simulink library "lib_fuel_converter"  (Simulink 4.00)
undefined symbols (not defined in the file): acc_mech_eff, acc_mech_pwr, acc_mech_trq, air_cp, amb_tmp, cyc_mph, ex_gas_cp, fc_acc_mass, fc_base_mass, fc_c2i_th_cond, fc_c_init_tmp, fc_cl2h_eff, fc_CO2_to_FUELgps, fc_cold, fc_cold_tmp, fc_cp, fc_ct_trq, fc_emisv, fc_ext_sarea, fc_fuel_den, fc_fuel_lhv, fc_h2x_th_cond, fc_h_air_flow, fc_h_cp, fc_h_init_tmp, fc_hood_emisv, fc_hood_sarea, fc_i2x_th_cond, fc_i_init_tmp, fc_inertia, fc_map_spd, fc_map_trq, fc_max_trq, fc_nn_model_name, fc_pwr_scale, fc_spd_scale, fc_trq_scale, fc_tstat, fc_x_init_tmp, fd_ratio, gb_num_init, gb_ratio, pow, vc_idle_spd, vc_key_on, veh_glider_mass, veh_mass, wh_radius
libraries: lib_fuel_converter x6, lib_etc x4
(part 4 of 4)

== system lib_fuel_converter/configurable subsystems/fuel use and EO emis/fc temp correct/fc temp correct Variable Correction Factors (Map Based)/CO factor cold-to-hot ==
  x0 : Inport  Port=1  LatchInput=off
  y0 : Inport  Port=2  LatchInput=off
  Mux : Mux  Inputs=2
      settings: DisplayOption=none
  S-function : S-Function  FunctionName=sftable2  Parameters=xindex, yindex, table  PortCounts=[]  SFunctionModules=''
  table out : Outport  Port=1  InitialOutput=0
  wires:
  Mux/1 -> S-function/1
  x0/1 -> Mux/1
  S-function/1 -> table out/1
  y0/1 -> Mux/2

== system lib_fuel_converter/configurable subsystems/fuel use and EO emis/fc temp correct/fc temp correct Variable Correction Factors (Map Based)/HC factor cold-to-hot ==
  x0 : Inport  Port=1  LatchInput=off
  y0 : Inport  Port=2  LatchInput=off
  Mux : Mux  Inputs=2
      settings: DisplayOption=none
  S-function : S-Function  FunctionName=sftable2  Parameters=xindex, yindex, table  PortCounts=[]  SFunctionModules=''
  table out : Outport  Port=1  InitialOutput=0
  wires:
  Mux/1 -> S-function/1
  x0/1 -> Mux/1
  S-function/1 -> table out/1
  y0/1 -> Mux/2

== system lib_fuel_converter/configurable subsystems/fuel use and EO emis/fc temp correct/fc temp correct Variable Correction Factors (Map Based)/NOx factor cold-to-hot ==
  x0 : Inport  Port=1  LatchInput=off
  y0 : Inport  Port=2  LatchInput=off
  Mux : Mux  Inputs=2
      settings: DisplayOption=none
  S-function : S-Function  FunctionName=sftable2  Parameters=xindex, yindex, table  PortCounts=[]  SFunctionModules=''
  table out : Outport  Port=1  InitialOutput=0
  wires:
  Mux/1 -> S-function/1
  x0/1 -> Mux/1
  S-function/1 -> table out/1
  y0/1 -> Mux/2

== system lib_fuel_converter/configurable subsystems/fuel use and EO emis/fc temp correct/fc temp correct Variable Correction Factors (Map Based)/PM factor cold-to-hot ==
  x0 : Inport  Port=1  LatchInput=off
  y0 : Inport  Port=2  LatchInput=off
  Mux : Mux  Inputs=2
      settings: DisplayOption=none
  S-function : S-Function  FunctionName=sftable2  Parameters=xindex, yindex, table  PortCounts=[]  SFunctionModules=''
  table out : Outport  Port=1  InitialOutput=0
  wires:
  Mux/1 -> S-function/1
  x0/1 -> Mux/1
  S-function/1 -> table out/1
  y0/1 -> Mux/2

== system lib_fuel_converter/configurable subsystems/fuel use and EO emis/fc temp correct/fc temp correct Variable Correction Factors (Map Based)/fuel factor cold-to-hot ==
  x0 : Inport  Port=1  LatchInput=off
  y0 : Inport  Port=2  LatchInput=off
  Mux : Mux  Inputs=2
      settings: DisplayOption=none
  S-function : S-Function  FunctionName=sftable2  Parameters=xindex, yindex, table  PortCounts=[]  SFunctionModules=''
  table out : Outport  Port=1  InitialOutput=0
  wires:
  Mux/1 -> S-function/1
  x0/1 -> Mux/1
  S-function/1 -> table out/1
  y0/1 -> Mux/2

== system lib_fuel_converter/configurable subsystems/fuel use and EO emis Neural Network Model/fc temp/fc mass heat flow/Block NOTES ==
  note: FUEL CONVERTER MASS HEAT LOSS
      | This block models the heat loss from a fuel converter (such as an IC engine).
      | Convection (as a function of vehicle speed), radiation, and conduction effects are included.
      | Engine cylinder (c), interior (i), exterior (x) and hood (h)
      | heat flows are estimated based on the temperatures from the previous iteration.

== system lib_fuel_converter/configurable subsystems/fuel use and EO emis Neural Network Model/fc temp/old fc coolant  temp. (C)/Block NOTES ==
  note: This block computes engine coolant temperature,
      | assuming that it asymptotically approaches its maximum
      | temperature when the engine is on, and asymptotically
      | approaches the ambient temperature when the engine
      | is off.  Temperatue rise rate is assumed to be a function
      | only of current engine coolant temperature, and the fall
      | rate is also a function of vehicle speed and ambient temperature.
      | There is no dependence on engine load or speed.

== system lib_fuel_converter/configurable subsystems/fuel use and EO emis Neural Network Model/fc temp correct/fc temp correct Constant Correction Factors (Equation Based)/Block NOTES ==
  note: This block determines actual fuel use and engine-out emissions
      | given the fully hot values and the engine coolant temperature.
      | The correlations used here were developed at NREL using
      | Hot and Cold Engine data collected
      | at Oak Ridge National Laboratory.

== system lib_fuel_converter/configurable subsystems/fuel use and EO emis Neural Network Model/fc temp correct/fc temp correct Variable Correction Factors (Map Based)/CO factor cold-to-hot ==
  x0 : Inport  Port=1  LatchInput=off
  y0 : Inport  Port=2  LatchInput=off
  Mux : Mux  Inputs=2
      settings: DisplayOption=none
  S-function : S-Function  FunctionName=sftable2  Parameters=xindex, yindex, table  PortCounts=[]  SFunctionModules=''
  table out : Outport  Port=1  InitialOutput=0
  wires:
  Mux/1 -> S-function/1
  x0/1 -> Mux/1
  S-function/1 -> table out/1
  y0/1 -> Mux/2

== system lib_fuel_converter/configurable subsystems/fuel use and EO emis Neural Network Model/fc temp correct/fc temp correct Variable Correction Factors (Map Based)/HC factor cold-to-hot ==
  x0 : Inport  Port=1  LatchInput=off
  y0 : Inport  Port=2  LatchInput=off
  Mux : Mux  Inputs=2
      settings: DisplayOption=none
  S-function : S-Function  FunctionName=sftable2  Parameters=xindex, yindex, table  PortCounts=[]  SFunctionModules=''
  table out : Outport  Port=1  InitialOutput=0
  wires:
  Mux/1 -> S-function/1
  x0/1 -> Mux/1
  S-function/1 -> table out/1
  y0/1 -> Mux/2

== system lib_fuel_converter/configurable subsystems/fuel use and EO emis Neural Network Model/fc temp correct/fc temp correct Variable Correction Factors (Map Based)/NOx factor cold-to-hot ==
  x0 : Inport  Port=1  LatchInput=off
  y0 : Inport  Port=2  LatchInput=off
  Mux : Mux  Inputs=2
      settings: DisplayOption=none
  S-function : S-Function  FunctionName=sftable2  Parameters=xindex, yindex, table  PortCounts=[]  SFunctionModules=''
  table out : Outport  Port=1  InitialOutput=0
  wires:
  Mux/1 -> S-function/1
  x0/1 -> Mux/1
  S-function/1 -> table out/1
  y0/1 -> Mux/2

== system lib_fuel_converter/configurable subsystems/fuel use and EO emis Neural Network Model/fc temp correct/fc temp correct Variable Correction Factors (Map Based)/PM factor cold-to-hot ==
  x0 : Inport  Port=1  LatchInput=off
  y0 : Inport  Port=2  LatchInput=off
  Mux : Mux  Inputs=2
      settings: DisplayOption=none
  S-function : S-Function  FunctionName=sftable2  Parameters=xindex, yindex, table  PortCounts=[]  SFunctionModules=''
  table out : Outport  Port=1  InitialOutput=0
  wires:
  Mux/1 -> S-function/1
  x0/1 -> Mux/1
  S-function/1 -> table out/1
  y0/1 -> Mux/2

== system lib_fuel_converter/configurable subsystems/fuel use and EO emis Neural Network Model/fc temp correct/fc temp correct Variable Correction Factors (Map Based)/fuel factor cold-to-hot ==
  x0 : Inport  Port=1  LatchInput=off
  y0 : Inport  Port=2  LatchInput=off
  Mux : Mux  Inputs=2
      settings: DisplayOption=none
  S-function : S-Function  FunctionName=sftable2  Parameters=xindex, yindex, table  PortCounts=[]  SFunctionModules=''
  table out : Outport  Port=1  InitialOutput=0
  wires:
  Mux/1 -> S-function/1
  x0/1 -> Mux/1
  S-function/1 -> table out/1
  y0/1 -> Mux/2
